simulink model "question_3"  (R2019a)
settings: Solver=ode4  StartTime=0.0  StopTime=50.0  FixedStep=0.001  RelTol=1e-3
settings Model: Creator=guima  LastModifiedBy=guima

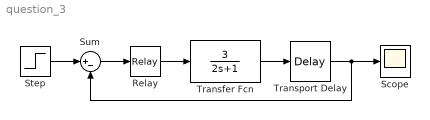
== system question_3 ==
  Relay : Relay  OnSwitchValue=0.1  OffSwitchValue=-0.1  OnOutputValue=5  OffOutputValue=-5
  Scope : Scope
  Step : Step  Time=eps  SampleTime=0
  Sum : Sum  Inputs=|+-
  Transfer Fcn : TransferFcn  Numerator=[3]  Denominator=[2 1]
  Transport Delay : TransportDelay  DelayTime=0.1
  wires:
  Sum/1 -> Relay/1
  Relay/1 -> Transfer Fcn/1
  Step/1 -> Sum/1
  Transfer Fcn/1 -> Transport Delay/1
  Transport Delay/1 -> Scope/1, Sum/2
